simulink model "understandingof_cotangentwave"  (R2024b)
settings: Solver=VariableStepAuto  StartTime=0.0  StopTime=25  MaxStep=0.001  RelTol=1e-3
settings Model: Creator=admin  LastModifiedBy=admin

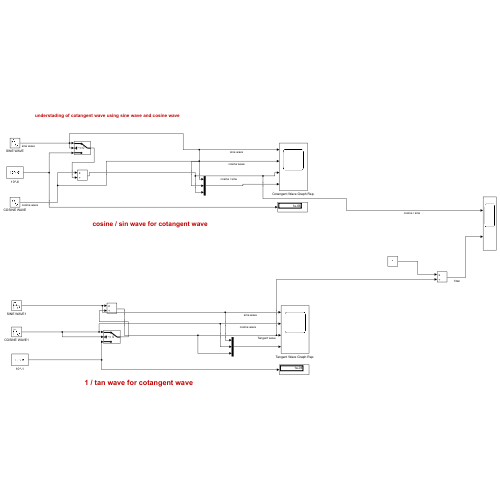
[thumbnail: Simulink's stored preview of the top-level diagram]
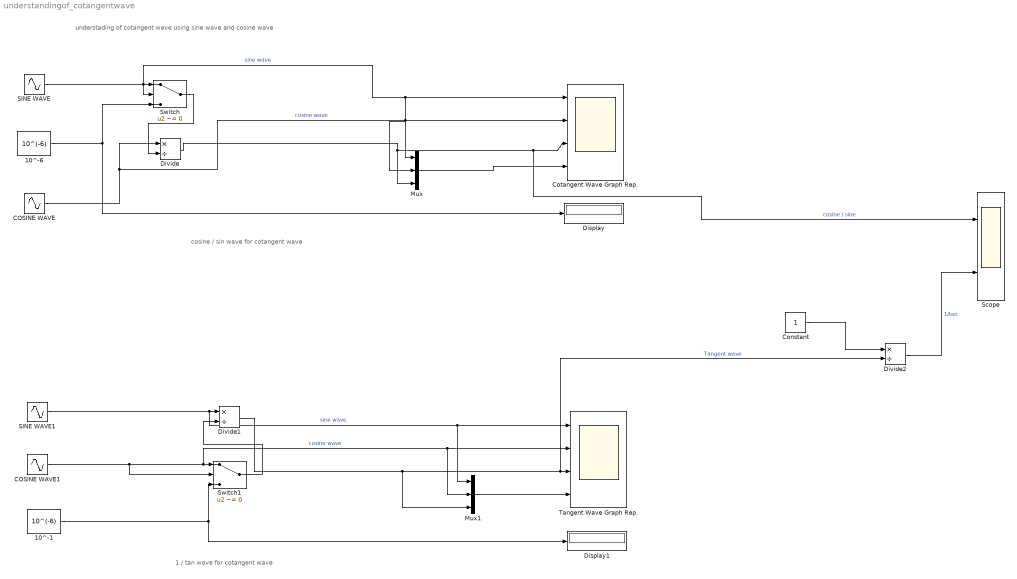
== system understandingof_cotangentwave ==
  note: 1 / tan wave for cotangent wave
  note: cosine / sin wave for cotangent wave
  note: understading of cotangent wave using sine wave and cosine wave
  10^-1 : Constant  Value=10^(-6)
  10^-6 : Constant  Value=10^(-6)
  COSINE WAVE : Sin  Phase=pi/2  SampleTime=0
  COSINE WAVE1 : Sin  Phase=pi/2  SampleTime=0
  Constant : Constant
  Cotangent Wave Graph Rep. : Scope  NumInputPorts=4
  Display : Display
  Display1 : Display
  Divide : Product  Inputs=*/
  Divide1 : Product  Inputs=*/
  Divide2 : Product  Inputs=*/
  Mux : Mux  Inputs=3
  Mux1 : Mux  Inputs=3
  SINE WAVE : Sin  SampleTime=0
  SINE WAVE1 : Sin  SampleTime=0
  Scope : Scope  NumInputPorts=2
  Switch : Switch  Criteria=u2 ~= 0  SaturateOnIntegerOverflow=off  InputSameDT=off
  Switch1 : Switch  Criteria=u2 ~= 0  SaturateOnIntegerOverflow=off  InputSameDT=off
  Tangent Wave Graph Rep. : Scope  NumInputPorts=4
  wires:
  10^-6/1 -> Display/1, Switch/3
  SINE WAVE/1 -> Switch/2, Switch/1, Mux/1, Cotangent Wave Graph Rep./1  "sine wave"
  COSINE WAVE/1 -> Mux/2, Cotangent Wave Graph Rep./2, Divide/1  "cosine wave"
  Switch/1 -> Divide/2
  Divide/1 -> Scope/1, Cotangent Wave Graph Rep./3, Mux/3  "cosine / sine"
  Mux/1 -> Cotangent Wave Graph Rep./4
  COSINE WAVE1/1 -> Switch1/2, Mux1/2, Tangent Wave Graph Rep./2, Switch1/1  "cosine wave"
  Divide1/1 -> Divide2/2, Tangent Wave Graph Rep./3, Mux1/3  "Tangent wave"
  Mux1/1 -> Tangent Wave Graph Rep./4
  Switch1/1 -> Divide1/2
  SINE WAVE1/1 -> Mux1/1, Tangent Wave Graph Rep./1, Divide1/1  "sine wave"
  10^-1/1 -> Display1/1, Switch1/3
  Constant/1 -> Divide2/1
  Divide2/1 -> Scope/2  "1/tan"
